simulink model "CIC_Decimator_Example"  (R2023a)
settings: Solver=VariableStepAuto  StartTime=0.0  StopTime=100  RelTol=1e-3
libraries: dspmlti4 x3
settings Model: Creator=Hasan  LastModifiedBy=Hasan
settings DebuggingCC: ParameterPrecisionLossMsg=none

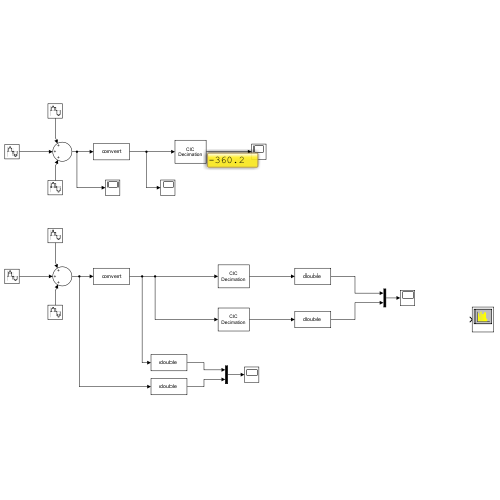
[thumbnail: Simulink's stored preview of the top-level diagram]
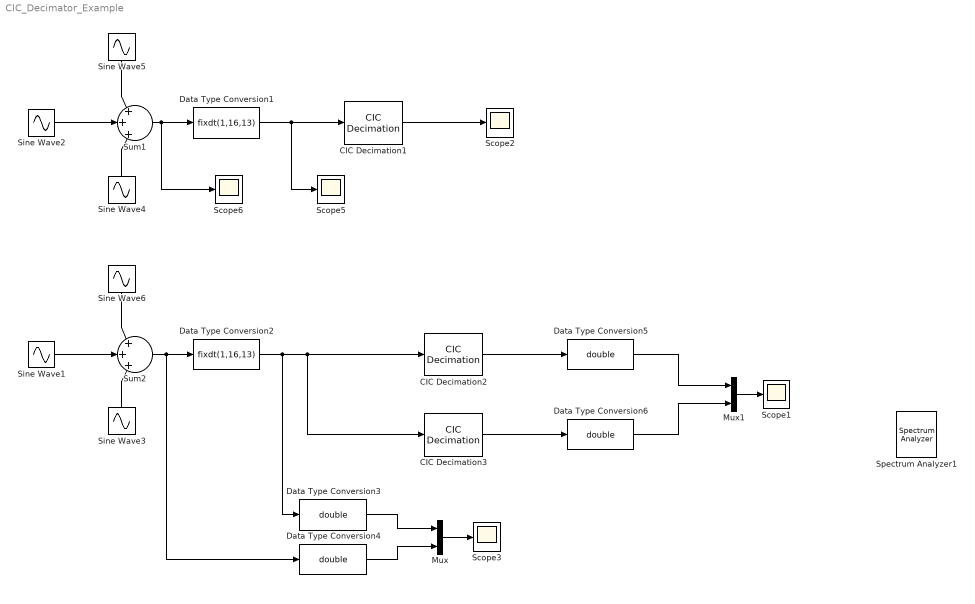
== system CIC_Decimator_Example ==
  CIC Decimation1 : dspmlti4/CIC Decimation  filtFrom=Dialog parameters  filtobj=CICDECIM  ftype=Decimator  R=10  M=1  N=3  filterInternals=Full precision  BPS=[16 16 16 16]  FLPS=0  outputWordLength=32  outputFracLength=0  launchFVT=off  framing=Maintain input frame rate  RateOptions=Allow multirate processing
  CIC Decimation2 : dspmlti4/CIC Decimation  filtFrom=Dialog parameters  filtobj=CICDECIM  ftype=Decimator  R=10  M=1  N=3  filterInternals=Full precision  BPS=[16 16 16 16]  FLPS=0  outputWordLength=32  outputFracLength=0  launchFVT=off  framing=Maintain input frame rate  RateOptions=Allow multirate processing
  CIC Decimation3 : dspmlti4/CIC Decimation  filtFrom=Dialog parameters  filtobj=CICDECIM  ftype=Decimator  R=10  M=1  N=3  filterInternals=Minimum section word lengths  BPS=[16 16 16 16]  FLPS=0  outputWordLength=12  outputFracLength=0  launchFVT=off  framing=Maintain input frame rate  RateOptions=Allow multirate processing
  Data Type Conversion1 : DataTypeConversion  OutDataTypeStr=fixdt(1,16,13)  SaturateOnIntegerOverflow=off  RndMeth=Floor
  Data Type Conversion2 : DataTypeConversion  OutDataTypeStr=fixdt(1,16,13)  SaturateOnIntegerOverflow=off  RndMeth=Floor
  Data Type Conversion{3..6} (4 alike) : DataTypeConversion  OutDataTypeStr=double  SaturateOnIntegerOverflow=off  RndMeth=Floor
  Mux : Mux  Inputs=2
  Mux1 : Mux  Inputs=2
  Scope{1..3,5..6} (5 alike) : Scope
  Sine Wave1 : Sin  Frequency=2*pi  SampleTime=1/1000
  Sine Wave2 : Sin  Frequency=2*pi  SampleTime=1/1000
  Sine Wave3 : Sin  Frequency=2*pi*5  SampleTime=1/1000
  Sine Wave4 : Sin  Frequency=2*pi*5  SampleTime=1/1000
  Sine Wave5 : Sin  Frequency=2*pi*50  SampleTime=1/1000
  Sine Wave6 : Sin  Frequency=2*pi*50  SampleTime=1/1000
  Spectrum Analyzer1 : SpectrumAnalyzer  WindowPosition=[368.000000,182.000000,800.000000,500.000000,]  ScopeFrameLocation=window  PlotAsTwoSidedSpectrum=off  YLimits=[-99.84683913,49.14753028]  ColorLimits=[-80 20]  SelectedToolstripTab=spectrumAnalyzerToolstrip.spectrumTab
  Sum1 : Sum  Inputs=|+|+|+|
  Sum2 : Sum  Inputs=|+|+|+|
  wires:
  Sine Wave2/1 -> Sum1/2
  Sine Wave4/1 -> Sum1/3
  Sine Wave5/1 -> Sum1/1
  Sum1/1 -> Scope6/1, Data Type Conversion1/1
  Data Type Conversion1/1 -> Scope5/1, CIC Decimation1/1
  CIC Decimation1/1 -> Scope2/1
  Data Type Conversion2/1 -> Data Type Conversion3/1, CIC Decimation3/1, CIC Decimation2/1
  Sine Wave6/1 -> Sum2/1
  Sine Wave1/1 -> Sum2/2
  Sine Wave3/1 -> Sum2/3
  Mux/1 -> Scope3/1
  Sum2/1 -> Data Type Conversion4/1, Data Type Conversion2/1
  Data Type Conversion4/1 -> Mux/2
  Data Type Conversion3/1 -> Mux/1
  CIC Decimation2/1 -> Data Type Conversion5/1
  CIC Decimation3/1 -> Data Type Conversion6/1
  Mux1/1 -> Scope1/1
  Data Type Conversion5/1 -> Mux1/1
  Data Type Conversion6/1 -> Mux1/2
